simulink subsystem "htx_fz_estimator"  (R2024b)
settings: Solver=VariableStepAuto  StartTime=0.0  StopTime=10.0  RelTol=1e-3
settings Model: Creator=lukec  LastModifiedBy=lukec

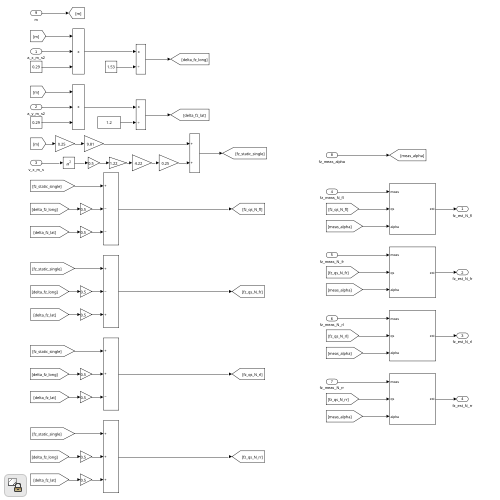
[thumbnail: Simulink's stored preview of the top-level diagram]
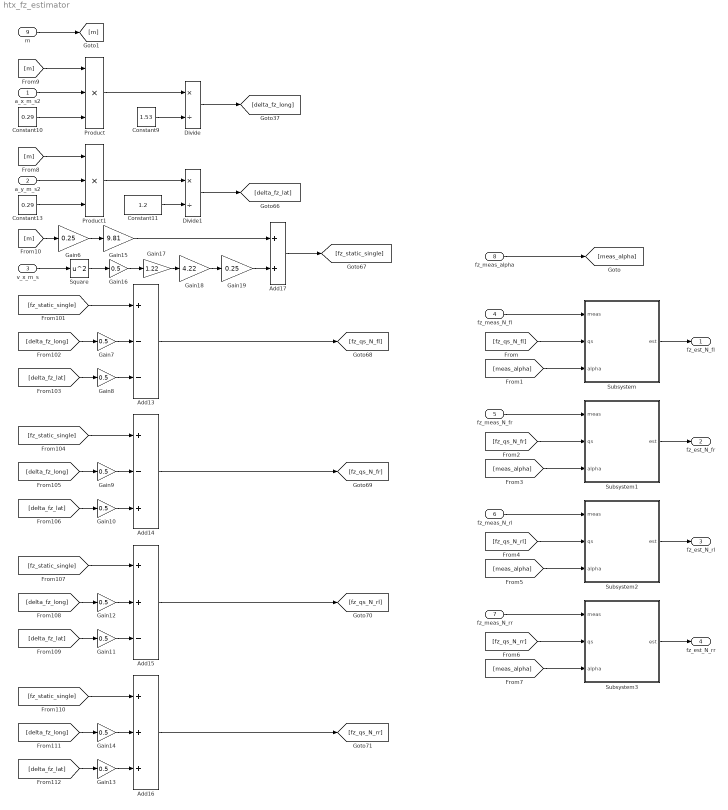
== system htx_fz_estimator ==
  a_x_m_s2 : Inport
  a_y_m_s2 : Inport  Port=2
  v_x_m_s : Inport  Port=3
  fz_meas_N_fl : Inport  Port=4
  fz_meas_N_fr : Inport  Port=5
  fz_meas_N_rl : Inport  Port=6
  fz_meas_N_rr : Inport  Port=7
  fz_meas_alpha : Inport  Port=8
  m : Inport  Port=9
  Add13 : Sum  Inputs=+--
  Add14 : Sum  Inputs=+-+
  Add15 : Sum  Inputs=++-
  Add16 : Sum  Inputs=+++
  Add17 : Sum
  Constant10 : Constant  Value=0.29
  Constant11 : Constant  Value=1.2
  Constant13 : Constant  Value=0.29
  Constant9 : Constant  Value=1.53
  Divide : Product  Inputs=*/
  Divide1 : Product  Inputs=*/
  Gain{7..14,16} (9 alike) : Gain  Gain=0.5
  Gain15 : Gain  Gain=9.81
  Gain17 : Gain  Gain=1.22
  Gain18 : Gain  Gain=4.22
  Gain19 : Gain  Gain=0.25
  Gain6 : Gain  Gain=0.25
  Product : Product  Inputs=3
  Product1 : Product  Inputs=3
  Square : Math  Operator=square
  Subsystem : Subsystem
  Subsystem1 : Subsystem
  Subsystem2 : Subsystem
  Subsystem3 : Subsystem
  fz_est_N_fl : Outport
  fz_est_N_fr : Outport  Port=2
  fz_est_N_rl : Outport  Port=3
  fz_est_N_rr : Outport  Port=4
  wires:
  [delta_fz_lat] -> Gain8/1
  Constant13/1 -> Product1/3
  [delta_fz_lat] -> Gain13/1
  [fz_static_single] -> Add14/1
  [delta_fz_long] -> Gain7/1
  Add15/1 -> [fz_qs_N_rl]
  Product1/1 -> Divide1/1
  [delta_fz_long] -> Gain12/1
  [delta_fz_lat] -> Gain10/1
  Gain6/1 -> Gain15/1
  [delta_fz_long] -> Gain14/1
  Constant9/1 -> Divide/2
  Add17/1 -> [fz_static_single]
  Gain14/1 -> Add16/2
  Gain9/1 -> Add14/2
  Gain12/1 -> Add15/2
  Gain17/1 -> Gain18/1
  [fz_static_single] -> Add16/1
  Constant11/1 -> Divide1/2
  v_x_m_s/1 -> Square/1
  Gain8/1 -> Add13/3
  Add13/1 -> [fz_qs_N_fl]
  Gain11/1 -> Add15/3
  [fz_static_single] -> Add15/1
  Gain19/1 -> Add17/2
  Gain16/1 -> Gain17/1
  a_x_m_s2/1 -> Product/2
  Add16/1 -> [fz_qs_N_rr]
  Add14/1 -> [fz_qs_N_fr]
  a_y_m_s2/1 -> Product1/2
  Divide1/1 -> [delta_fz_lat]
  Gain7/1 -> Add13/2
  Gain10/1 -> Add14/3
  Divide/1 -> [delta_fz_long]
  [fz_static_single] -> Add13/1
  [delta_fz_long] -> Gain9/1
  [delta_fz_lat] -> Gain11/1
  Square/1 -> Gain16/1
  Gain18/1 -> Gain19/1
  Constant10/1 -> Product/3
  Gain13/1 -> Add16/3
  Gain15/1 -> Add17/1
  Product/1 -> Divide/1
  fz_meas_alpha/1 -> [meas_alpha]
  fz_meas_N_fl/1 -> Subsystem/1(meas)
  [fz_qs_N_fl] -> Subsystem/2(qs)
  [meas_alpha] -> Subsystem/3(alpha)
  Subsystem/1(est) -> fz_est_N_fl/1
  Subsystem1/1(est) -> fz_est_N_fr/1
  [meas_alpha] -> Subsystem1/3(alpha)
  [fz_qs_N_fr] -> Subsystem1/2(qs)
  [fz_qs_N_rl] -> Subsystem2/2(qs)
  [meas_alpha] -> Subsystem2/3(alpha)
  Subsystem2/1(est) -> fz_est_N_rl/1
  Subsystem3/1(est) -> fz_est_N_rr/1
  [meas_alpha] -> Subsystem3/3(alpha)
  [fz_qs_N_rr] -> Subsystem3/2(qs)
  fz_meas_N_rr/1 -> Subsystem3/1(meas)
  fz_meas_N_rl/1 -> Subsystem2/1(meas)
  fz_meas_N_fr/1 -> Subsystem1/1(meas)
  m/1 -> [m]
  [m] -> Product1/1
  [m] -> Product/1
  [m] -> Gain6/1

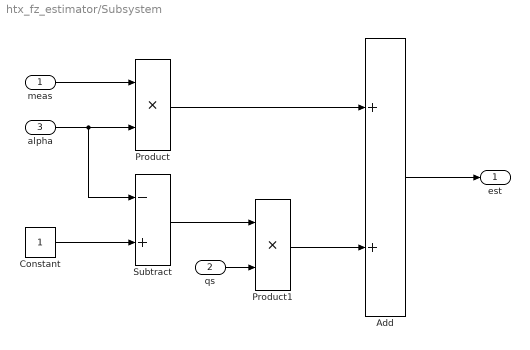
== system htx_fz_estimator/Subsystem ==
  meas : Inport
  qs : Inport  Port=2
  alpha : Inport  Port=3
  Add : Sum
  Constant : Constant
  Product : Product
  Product1 : Product
  Subtract : Sum  Inputs=-+
  est : Outport
  wires:
  Add/1 -> est/1
  Product1/1 -> Add/2
  qs/1 -> Product1/2
  Subtract/1 -> Product1/1
  Constant/1 -> Subtract/2
  Product/1 -> Add/1
  alpha/1 -> Product/2, Subtract/1
  meas/1 -> Product/1

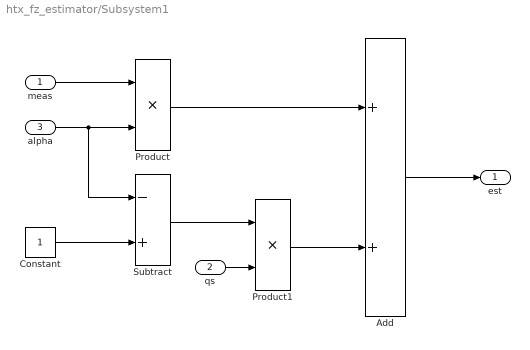
== system htx_fz_estimator/Subsystem1 ==
  meas : Inport
  qs : Inport  Port=2
  alpha : Inport  Port=3
  Add : Sum
  Constant : Constant
  Product : Product
  Product1 : Product
  Subtract : Sum  Inputs=-+
  est : Outport
  wires:
  meas/1 -> Product/1
  alpha/1 -> Subtract/1, Product/2
  Product/1 -> Add/1
  Constant/1 -> Subtract/2
  Subtract/1 -> Product1/1
  qs/1 -> Product1/2
  Product1/1 -> Add/2
  Add/1 -> est/1

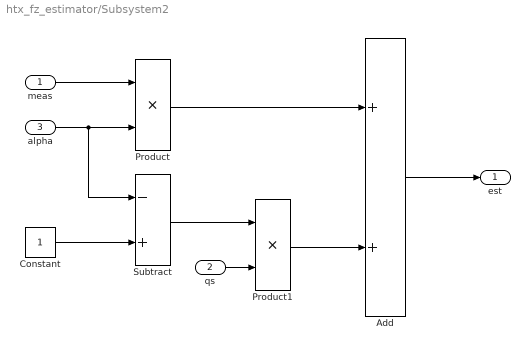
== system htx_fz_estimator/Subsystem2 ==
  meas : Inport
  qs : Inport  Port=2
  alpha : Inport  Port=3
  Add : Sum
  Constant : Constant
  Product : Product
  Product1 : Product
  Subtract : Sum  Inputs=-+
  est : Outport
  wires:
  Add/1 -> est/1
  Product1/1 -> Add/2
  qs/1 -> Product1/2
  Subtract/1 -> Product1/1
  Constant/1 -> Subtract/2
  Product/1 -> Add/1
  alpha/1 -> Product/2, Subtract/1
  meas/1 -> Product/1

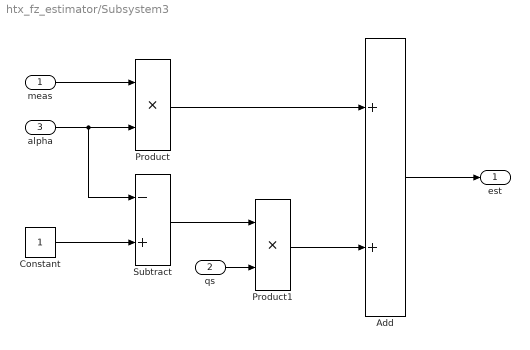
== system htx_fz_estimator/Subsystem3 ==
  meas : Inport
  qs : Inport  Port=2
  alpha : Inport  Port=3
  Add : Sum
  Constant : Constant
  Product : Product
  Product1 : Product
  Subtract : Sum  Inputs=-+
  est : Outport
  wires:
  meas/1 -> Product/1
  alpha/1 -> Subtract/1, Product/2
  Product/1 -> Add/1
  Constant/1 -> Subtract/2
  Subtract/1 -> Product1/1
  qs/1 -> Product1/2
  Product1/1 -> Add/2
  Add/1 -> est/1
